simulink model "flexlink_exp"  (R2022a)
settings: Solver=ode1  StartTime=0.0  StopTime=10  FixedStep=0.002  RelTol=1e-3  EnableMultiTasking=on
values from neighbouring files (symbols this model uses):
  K = [13.0384048104 -17.2586438179 1.31984719989 -0.0460779069804]    [LQRFlexibleJoint.mat]    (also in LQRFlexibleLink.mat = [12.6491106407 -13.4510037877 1.04396559995 0.0309235004795]; PDControllerA.mat = [4.74 0 0.2133 0]; PDControllerB.mat = [4.74 4.74 0.2133 0.2133]; config_flexjoint.m = aK(SPRING))
  K_ENC = 0.00153398078789    [LQRFlexibleJoint.mat]    (also in LQRFlexibleLink.mat; PDControllerA.mat; PDControllerB.mat; config_servo_exp.m = 0)
  K_GAGE = 0.0526315789474    [LQRFlexibleLink.mat]    (also in config_flexgage_exp.m)
  VMAX_UPM = 15    [LQRFlexibleJoint.mat]    (also in LQRFlexibleLink.mat = 24; PDControllerA.mat; PDControllerB.mat; config_servo_exp.m = 0)
  wcf_1 = 207.345115137    [LQRFlexibleJoint.mat]    (also in LQRFlexibleLink.mat = 100.530964915; PDControllerA.mat; PDControllerB.mat; setup_flexjoint_exp.m)
  wcf_2 = 207.345115137    [LQRFlexibleJoint.mat]    (also in LQRFlexibleLink.mat = 18.8495559215; PDControllerA.mat; PDControllerB.mat; setup_flexjoint_exp.m)
undefined symbols (not defined in the file or in its folder): HIL, qc_get_step_size
libraries: quarc_library x5, simulink_extras x4
settings Model: ExtModeTrigDuration=10000  Creator=17stf1  LastModifiedBy=17stf1
settings SolverCC: AlgebraicLoopSolver=TrustRegion  PositivePriorityOrder=on
settings DataIOCC: ReturnWorkspaceOutputs=off
settings DebuggingCC: UnconnectedInputMsg=warning  UnconnectedOutputMsg=warning  UnconnectedLineMsg=warning  SFMachineParentedDataDiag=warning  ArithmeticOperatorsInVariantConditions=warning
settings SFSimCC: SimUseLocalCustomCode=off  CustomCodeUndefinedFunction=UseInterfaceOnly
settings RTWCC: Description=QUARC Win64 Target Using Toolchain  SystemTargetFile=quarc_win64.tlc  TemplateMakefile=quarc_default_tmf  RTWUseLocalCustomCode=off  Toolchain=QUARC win64 | nmake (64-bit Windows)  BuildConfiguration=Faster Runs  DLArmComputeVersion=19.05
settings CodeAppCC: StateflowObjectComments=on
settings STFCustomTargetCC: TargetLangStandard=C99 (ISO)  ConcurrentExecutionCompliant=on  UseToolchainInfoCompliant=on  SystemTargetFile=quarc_win64.tlc
settings GRTTargetCC: ParMdlRefBuildCompliant=off  CompOptLevelCompliant=off  CombineOutputUpdateFcns=off  MatFileLogging=off  CPPClassGenCompliant=off  GRTInterface=on  ExtMode=on  ExtModeMexFile=quarc_comm
settings ConfigComp: CovMetricSettings=dswe

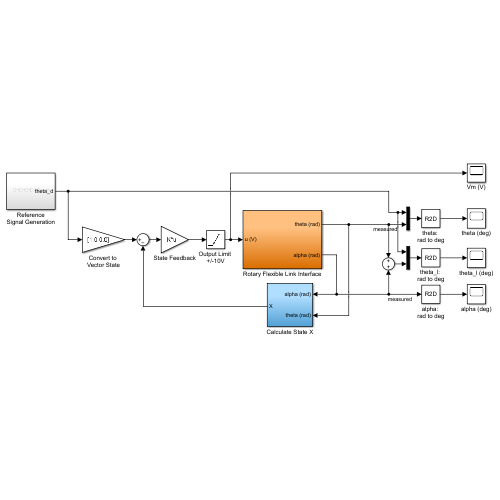
[thumbnail: Simulink's stored preview of the top-level diagram]
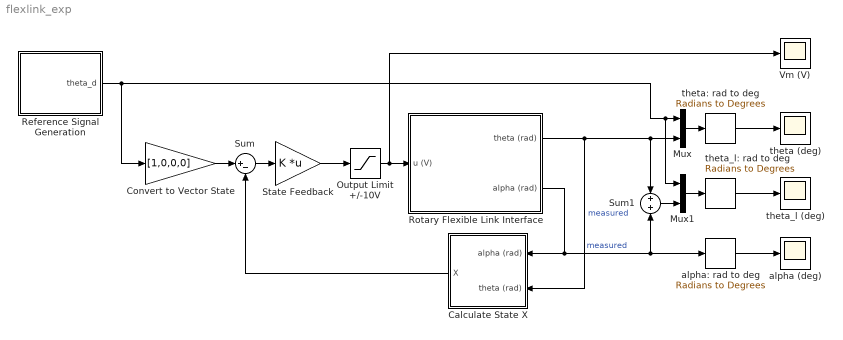
== system flexlink_exp ==
  Calculate State X : Subsystem
  Convert to Vector State : Gain  Gain=[1,0,0,0]
  Mux : Mux  Inputs=2
  Mux1 : Mux  Inputs=2
  Output Limit +/-10V : Saturate  UpperLimit=10  LowerLimit=-10
  Reference Signal Generation : Subsystem
  Rotary Flexible Link Interface : Subsystem
  State Feedback : Gain  Gain=K  Multiplication=Matrix(K*u)  SaturateOnIntegerOverflow=on  OutDataTypeStr=Inherit: Same as input  ParamDataTypeStr=Inherit: Same as input
  Sum : Sum  Inputs=|+-
  Sum1 : Sum
  Vm (V) : Scope
  alpha (deg) : Scope
  alpha: rad to deg : simulink_extras/Transformations/Radians to Degrees
  theta (deg) : Scope
  theta: rad to deg : simulink_extras/Transformations/Radians to Degrees
  theta_l (deg) : Scope
  theta_l: rad to deg : simulink_extras/Transformations/Radians to Degrees
  wires:
  theta: rad to deg/1 -> theta (deg)/1
  Mux1/1 -> theta_l: rad to deg/1
  Sum/1 -> State Feedback/1
  Output Limit +/-10V/1 -> Rotary Flexible Link Interface/1(u (V)), Vm (V)/1
  Reference Signal Generation/1(theta_d) -> Mux1/1, Mux/1, Convert to Vector State/1
  theta_l: rad to deg/1 -> theta_l (deg)/1
  Sum1/1 -> Mux1/2
  Rotary Flexible Link Interface/1(theta (rad)) -> Calculate State X/2(theta (rad)), Sum1/1, Mux/2  "measured"
  Convert to Vector State/1 -> Sum/1
  Mux/1 -> theta: rad to deg/1
  alpha: rad to deg/1 -> alpha (deg)/1
  State Feedback/1 -> Output Limit +/-10V/1
  Rotary Flexible Link Interface/2(alpha (rad)) -> Sum1/2, alpha: rad to deg/1, Calculate State X/1(alpha (rad))  "measured"
  Calculate State X/1(X) -> Sum/2

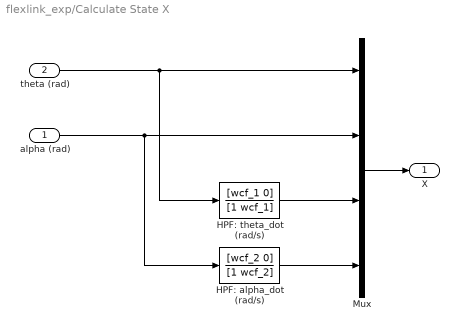
== system flexlink_exp/Calculate State X ==
  alpha (rad) : Inport
  theta (rad) : Inport  Port=2
  HPF: alpha_dot (rad/s) : TransferFcn  Numerator=[wcf_2 0]  Denominator=[1 wcf_2]
  HPF: theta_dot (rad/s) : TransferFcn  Numerator=[wcf_1 0]  Denominator=[1 wcf_1]
  Mux : Mux
  X : Outport  VectorParamsAs1DForOutWhenUnconnected=off
  wires:
  HPF: alpha_dot (rad/s)/1 -> Mux/4
  HPF: theta_dot (rad/s)/1 -> Mux/3
  theta (rad)/1 -> HPF: theta_dot (rad/s)/1, Mux/1
  Mux/1 -> X/1
  alpha (rad)/1 -> HPF: alpha_dot (rad/s)/1, Mux/2

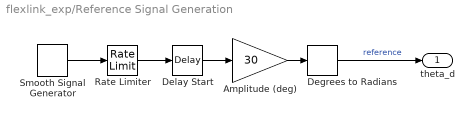
== system flexlink_exp/Reference Signal Generation ==
  Amplitude (deg) : Gain  Gain=30  SaturateOnIntegerOverflow=on  OutDataTypeStr=Inherit: Same as input  ParamDataTypeStr=Inherit: Same as input
  Degrees to Radians : simulink_extras/Transformations/Degrees to Radians
  Delay Start : TransportDelay  DelayTime=0.2  BufferSize=0.2/qc_get_step_size
  Rate Limiter : RateLimiter  RisingSlewLimit=100  FallingSlewLimit=-100  SampleTimeMode=inherited
  Smooth Signal Generator : quarc_library/Sources/Signals/Smooth Signal Generator  signal_type=Square  source=Internal (dialog parameters)  amplitude=1  frequency=0.25  initial_phase=0  sample_time=qc_get_step_size  output_cos=off
      settings: SourceProductName=QUARC Targets
  theta_d : Outport
  wires:
  Delay Start/1 -> Amplitude (deg)/1
  Amplitude (deg)/1 -> Degrees to Radians/1
  Rate Limiter/1 -> Delay Start/1
  Smooth Signal Generator/1 -> Rate Limiter/1
  Degrees to Radians/1 -> theta_d/1  "reference"

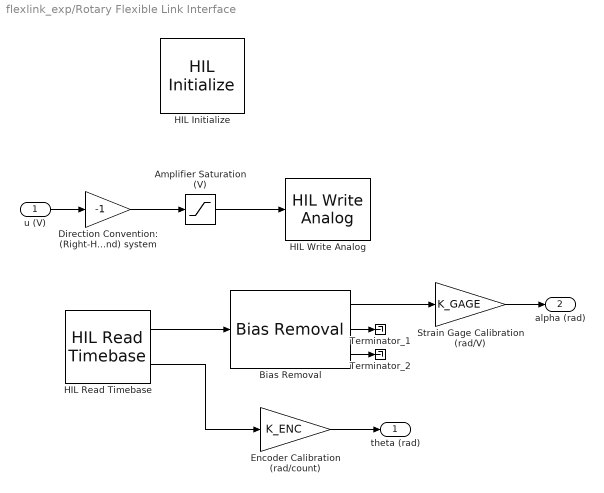
== system flexlink_exp/Rotary Flexible Link Interface ==
  u (V) : Inport
  Amplifier Saturation (V) : Saturate  UpperLimit=VMAX_UPM  LowerLimit=-VMAX_UPM
  Bias Removal : quarc_library/Discrete/Bias Removal  start_time=0  end_time=0.1  switch_id=0  sample_time=qc_get_step_size
      settings: SourceProductName=QUARC Targets
  Direction Convention: (Right-Hand) system : Gain  Gain=-1  SaturateOnIntegerOverflow=on  OutDataTypeStr=Inherit: Same as input  ParamDataTypeStr=Inherit: Same as input
  Encoder Calibration (rad/count) : Gain  Gain=K_ENC  SaturateOnIntegerOverflow=on  OutDataTypeStr=Inherit: Same as input  ParamDataTypeStr=Inherit: Same as input
  HIL Initialize : quarc_library/Data Acquisition/Generic/Configuration/HIL Initialize  object_name=HIL-1  board_type=q2_usb  board_number=0  board_options=d0=digital;d1=digital;led=auto;update_rate=normal;decimation=1  exclusive=off  active=on  hardware_clocks=[0]  clock_modes=[]  initial_clock_frequencies=[]  set_clock_params_at_start=off  set_clock_params_at_switch_in=off  set_clock_frequencies_at_start=off  set_clock_frequencies_at_switch_in=off  analog_input_channels=[0:1]  analog_input_configurations=[]  analog_input_maximums=10  analog_input_minimums=-10  set_analog_input_params_at_start=on  set_analog_input_params_at_switch_in=off  analog_output_channels=[0:1]  analog_output_maximums=10  analog_output_minimums=-10  initial_analog_outputs=[0]  final_analog_outputs=[0]  watchdog_analog_outputs=0  set_analog_output_params_at_start=on  set_analog_output_params_at_switch_in=off  set_analog_outputs_at_start=on  set_analog_outputs_at_switch_in=off  set_analog_outputs_at_terminate=on  set_analog_outputs_at_switch_out=off  set_analog_outputs_on_watchdog=off  digital_input_channels=[]  digital_output_channels=[]  digital_output_configuration=[]  initial_digital_outputs=[1]  final_digital_outputs=[1]  watchdog_digital_outputs=[1]  set_digital_output_params_at_start=off  set_digital_output_params_at_switch_in=off  set_digital_outputs_at_start=on  set_digital_outputs_at_switch_in=off  set_digital_outputs_at_terminate=on  set_digital_outputs_at_switch_out=off  set_digital_outputs_on_watchdog=off  encoder_channels=[0:1]  quadrature=[4]  encoder_filter_frequency=[]  initial_encoder_counts=[0]  set_encoder_params_at_start=on  set_encoder_params_at_switch_in=off  set_encoder_counts_at_start=on  set_encoder_counts_at_switch_in=off  pwm_channels=[]  pwm_modes=[0]  pwm_frequency=1/0.020  pwm_configuration=[]  pwm_alignment=[]  pwm_polarity=[]  pwm_leading_deadband=[]  pwm_trailing_deadband=[]  initial_pwm_outputs=[0]  final_pwm_outputs=[0]  watchdog_pwm_outputs=[0]  set_pwm_params_at_start=on  set_pwm_params_at_switch_in=off  set_pwm_outputs_at_start=on  set_pwm_outputs_at_switch_in=off  set_pwm_outputs_at_terminate=on  set_pwm_outputs_at_switch_out=off  set_pwm_outputs_on_watchdog=off  other_output_channels=[]  initial_other_outputs=[]  final_other_outputs=[]  watchdog_other_outputs=[]  set_other_outputs_at_start=off  set_other_outputs_at_switch_in=off  set_other_outputs_at_terminate=off  set_other_outputs_at_switch_out=off  set_other_outputs_on_watchdog=off
  HIL Read Timebase : quarc_library/Data Acquisition/Generic/Timebases/HIL Read Timebase  object_name=HIL-1  clock=0  analog_channels=[0]  encoder_channels=[0]  digital_channels=[]  other_channels=[]  active=on  vector_output=off  data_type_mode=Inherit via back propagation  encoder_data_type=double  digital_data_type=boolean  overflow_mode=Error on overflow  samples_in_buffer=max(ceil(1/qc_get_step_size), 1)
  HIL Write Analog : quarc_library/Data Acquisition/Generic/Immediate I//O/HIL Write Analog  object_name=HIL-1  channels=0  sample_time=-1  active=on  vector_input=off
  Strain Gage Calibration (rad/V) : Gain  Gain=K_GAGE  SaturateOnIntegerOverflow=on  OutDataTypeStr=Inherit: Same as input  ParamDataTypeStr=Inherit: Same as input
  Terminator_1 : Terminator
  Terminator_2 : Terminator
  theta (rad) : Outport  VectorParamsAs1DForOutWhenUnconnected=off
  alpha (rad) : Outport  Port=2  VectorParamsAs1DForOutWhenUnconnected=off
  wires:
  Amplifier Saturation (V)/1 -> HIL Write Analog/1
  u (V)/1 -> Direction Convention: (Right-Hand) system/1
  HIL Read Timebase/2 -> Encoder Calibration (rad/count)/1
  Direction Convention: (Right-Hand) system/1 -> Amplifier Saturation (V)/1
  Encoder Calibration (rad/count)/1 -> theta (rad)/1
  Bias Removal/2 -> Terminator_1/1
  HIL Read Timebase/1 -> Bias Removal/1
  Bias Removal/1 -> Strain Gage Calibration (rad/V)/1
  Strain Gage Calibration (rad/V)/1 -> alpha (rad)/1
  Bias Removal/3 -> Terminator_2/1
